simulink model "model_1"  (R2023b)
settings: Solver=VariableStepAuto  StartTime=0.0  StopTime=10.0  RelTol=1e-3
settings Model: Creator=pavig  LastModifiedBy=pavig

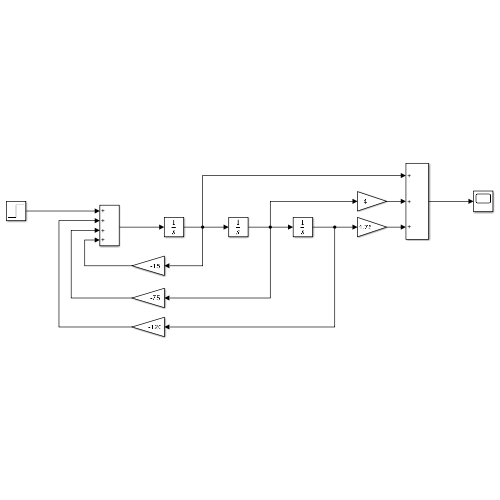
[thumbnail: Simulink's stored preview of the top-level diagram]
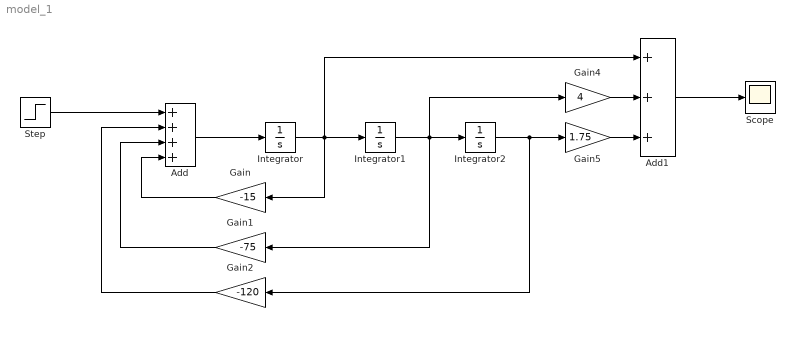
== system model_1 ==
  Add : Sum  Inputs=++++
  Add1 : Sum  Inputs=+++
  Gain : Gain  Gain=-15
  Gain1 : Gain  Gain=-75
  Gain2 : Gain  Gain=-120
  Gain4 : Gain  Gain=4
  Gain5 : Gain  Gain=1.75
  Integrator : Integrator
  Integrator1 : Integrator
  Integrator2 : Integrator
  Scope : Scope
  Step : Step  After=20  SampleTime=2
  wires:
  Integrator1/1 -> Gain1/1, Integrator2/1, Gain4/1
  Add/1 -> Integrator/1
  Step/1 -> Add/1
  Gain/1 -> Add/4
  Gain1/1 -> Add/3
  Gain2/1 -> Add/2
  Integrator2/1 -> Gain2/1, Gain5/1
  Gain5/1 -> Add1/3
  Gain4/1 -> Add1/2
  Integrator/1 -> Gain/1, Integrator1/1, Add1/1
  Add1/1 -> Scope/1
